simulink model "dPendDisUKF"  (Simulink 7.0)
settings: Solver=ode4  StartTime=0.0  StopTime=20  FixedStep=ts  RelTol=1e-3
InitFcn:
  | %dPendInit;
undefined symbols (not defined in the file): a, accel, B, b, c, c1, c2, d, g, l1, m, m1, m2, magnitude, n, p, P0, Qu, r1, r2, Ru, ts, W, WM, X0
libraries: simulink x4
settings Model: Creator=raje_ra  LastModifiedBy=vector  BufferReuse=off
settings OptimizationCC: OptimizeBlockIOStorage=off  BufferReuse=off  ExpressionFolding=off  LocalBlockOutputs=off

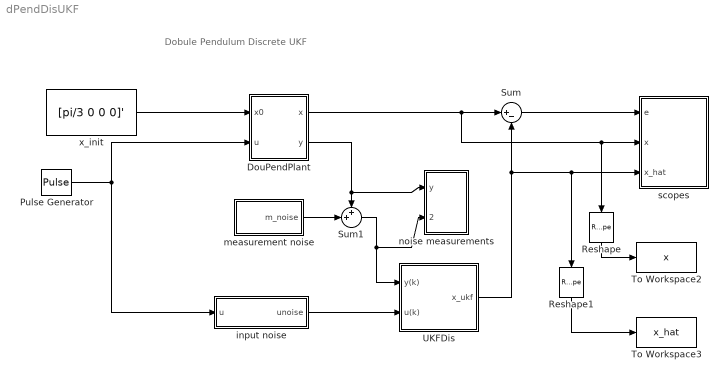
== system dPendDisUKF ==
  note: Dobule Pendulum Discrete UKF
  DouPendPlant : Subsystem
  Pulse Generator : DiscretePulseGenerator  PulseType=Time based  Amplitude=0.001  Period=1  PulseWidth=50
  Reshape : Reshape  Orientation=down
  Reshape1 : Reshape  Orientation=down
  Sum : Sum  Inputs=|+-  OutDataType=sfix(16)  OutScaling=2^0
  Sum1 : Sum  Inputs=++|  OutDataType=sfix(16)  OutScaling=2^0
  To Workspace2 : ToWorkspace  VariableName=x  SampleTime=-1  SaveFormat=Structure With Time
  To Workspace3 : ToWorkspace  VariableName=x_hat  SampleTime=-1  SaveFormat=Structure With Time
  UKFDis : Subsystem
  input noise : Subsystem
  measurement noise : Subsystem
  noise measurements : Subsystem
  scopes : Subsystem
  x_init : Constant  Value=[pi/3 0 0 0]'  VectorParams1D=off  OutDataType=sfix(16)  OutScaling=2^0
  wires:
  x_init/1 -> DouPendPlant/1(x0)
  DouPendPlant/1(x) -> Sum/1, scopes/2(x), Reshape/1
  UKFDis/1(x_ukf) -> Sum/2, scopes/3(x_hat), Reshape1/1
  Sum/1 -> scopes/1(e)
  Pulse Generator/1 -> DouPendPlant/2(u), input noise/1(u)
  DouPendPlant/2(y) -> Sum1/1, noise measurements/1(y)
  Sum1/1 -> UKFDis/1(y(k)), noise measurements/2(ynoise)
  measurement noise/1(m_noise) -> Sum1/2
  input noise/1(unoise) -> UKFDis/2(u(k))
  Reshape/1 -> To Workspace2/1
  Reshape1/1 -> To Workspace3/1

== system dPendDisUKF/DouPendPlant ==
  x0 : Inport
  u : Inport  Port=2
  F(x) : Subsystem
  Integrator1 : Integrator  InitialConditionSource=external  InitialCondition=[pi/3,-pi/3]'
  Measurements : Subsystem
  x : Outport  OutDataType=sfix(16)  OutScaling=2^0
  y : Outport  Port=2  OutDataType=sfix(16)  OutScaling=2^0
  wires:
  u/1 -> Measurements/2(u), F(x)/2(u)
  F(x)/1(x_dot) -> Integrator1/1
  Integrator1/1 -> x/1, F(x)/1(x), Measurements/1(x)  "x"
  x0/1 -> Integrator1/2
  Measurements/1(y) -> y/1

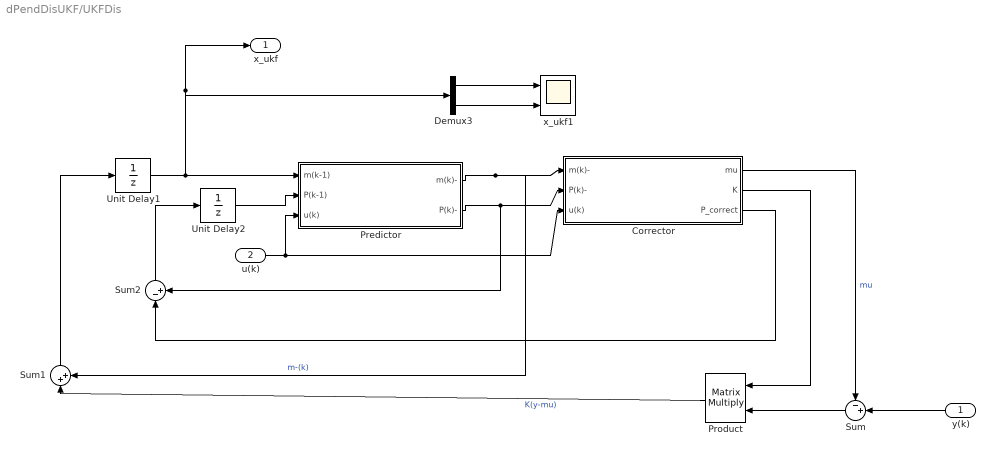
== system dPendDisUKF/UKFDis ==
  y(k) : Inport  Orientation=left
  u(k) : Inport  Port=2
  Corrector : Subsystem
  Demux3 : Demux  Outputs=2
  Predictor : Subsystem
  Product : Product  Orientation=left  Multiplication=Matrix(*)  OutDataType=sfix(16)  OutScaling=2^0  RndMeth=Zero
  Sum : Sum  Orientation=left  Inputs=-+|  OutDataType=sfix(16)  OutScaling=2^0
  Sum1 : Sum  Orientation=up  Inputs=|++  OutDataType=sfix(16)  OutScaling=2^0
  Sum2 : Sum  Orientation=up  Inputs=|-+  OutDataType=sfix(16)  OutScaling=2^0
  Unit Delay1 : UnitDelay  X0=X0  SampleTime=-1
  Unit Delay2 : UnitDelay  X0=P0  SampleTime=-1
  x_ukf1 : Scope  NumInputPorts=2
      settings: TimeRange=30  YMin=-15~-10  YMax=15~50  SaveName=ScopeData2
  x_ukf : Outport  OutDataType=sfix(16)  OutScaling=2^0
  wires:
  Sum2/1 -> Unit Delay2/1
  Corrector/3(P_correct) -> Sum2/1
  Unit Delay2/1 -> Predictor/2(P(k-1))
  Product/1 -> Sum1/1  "K(y-mu)"
  Sum/1 -> Product/2
  y(k)/1 -> Sum/2
  Corrector/2(K) -> Product/1
  Corrector/1(mu) -> Sum/1  "mu"
  Predictor/2(P(k)-) -> Sum2/2, Corrector/2(P(k)-)
  Predictor/1(m(k)-) -> Sum1/2, Corrector/1(m(k)-)  "m-(k)"
  Unit Delay1/1 -> Predictor/1(m(k-1)), x_ukf/1, Demux3/1
  Sum1/1 -> Unit Delay1/1
  Demux3/2 -> x_ukf1/2
  Demux3/1 -> x_ukf1/1
  u(k)/1 -> Predictor/3(u(k)), Corrector/3(u(k))

== system dPendDisUKF/input noise ==
  u : Inport
  Band-Limited White Noise : simulink/Sources/Band-Limited White Noise  SystemSampleTime=-1  Cov=[1e-6]  Ts=ts  seed=[23341]
  Sum2 : Sum  Inputs=++|  OutDataType=sfix(16)  OutScaling=2^0
  To Workspace2 : ToWorkspace  VariableName=Q_in  SampleTime=-1  SaveFormat=Array
  unoise : Outport
  wires:
  Sum2/1 -> unoise/1
  u/1 -> Sum2/2
  Band-Limited White Noise/1 -> To Workspace2/1, Sum2/1

== system dPendDisUKF/measurement noise ==
  Band-Limited White Noise - gyro : simulink/Sources/Band-Limited White Noise  SystemSampleTime=-1  Cov=[1e-7]  Ts=ts  seed=[23341]
  Band-Limited White Noise- q,dq : simulink/Sources/Band-Limited White Noise  SystemSampleTime=-1  Cov=[1e-9]  Ts=ts  seed=[23341]
  Band-Limited White Noise-IMU : simulink/Sources/Band-Limited White Noise  SystemSampleTime=-1  Cov=[1e-5]  Ts=ts  seed=[23341]
  Mux : Mux  Inputs=5
  To Workspace : ToWorkspace  VariableName=R_in  SampleTime=-1  SaveFormat=Array
  m_noise : Outport
  wires:
  Band-Limited White Noise-IMU/1 -> Mux/5, Mux/4
  Band-Limited White Noise - gyro/1 -> Mux/3
  Mux/1 -> To Workspace/1, m_noise/1
  Band-Limited White Noise- q,dq/1 -> Mux/2, Mux/1

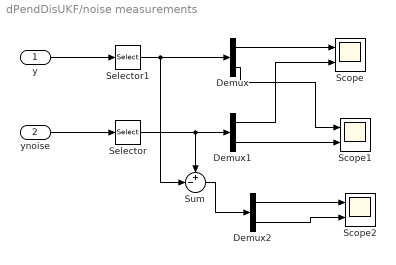
== system dPendDisUKF/noise measurements ==
  y : Inport
  ynoise : Inport  Port=2
  Demux : Demux  Outputs=2
  Demux1 : Demux  Outputs=2
  Demux2 : Demux  Outputs=2
  Scope : Scope  NumInputPorts=2
      settings: YMin=-60~-60  YMax=180~180
  Scope1 : Scope  NumInputPorts=2
      settings: YMin=-60~-60  YMax=180~180  SaveName=ScopeData5
  Scope2 : Scope  NumInputPorts=2
      settings: YMin=-60~-60  YMax=180~180  SaveName=ScopeData6
  Selector : Selector  InputPortWidth=5  IndexOptions=Index vector (dialog)  Indices=[1,2]  OutputSizes=1
  Selector1 : Selector  InputPortWidth=5  IndexOptions=Index vector (dialog)  Indices=[1,2]  OutputSizes=1
  Sum : Sum  Inputs=+-|  OutDataType=sfix(16)  OutScaling=2^0
  wires:
  Demux2/2 -> Scope2/2
  Demux2/1 -> Scope2/1
  Demux1/2 -> Scope1/2
  Demux/2 -> Scope1/1
  Demux1/1 -> Scope/2
  Demux/1 -> Scope/1
  Sum/1 -> Demux2/1
  Selector/1 -> Sum/1, Demux1/1
  Selector1/1 -> Sum/2, Demux/1
  ynoise/1 -> Selector/1
  y/1 -> Selector1/1

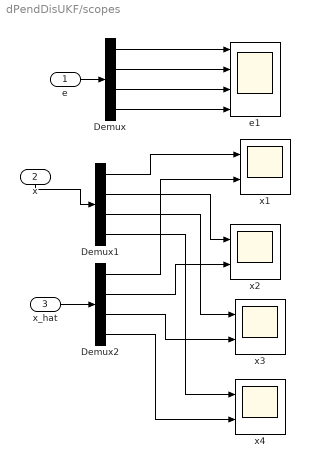
== system dPendDisUKF/scopes ==
  e : Inport
  x : Inport  Orientation=down  Port=2
  x_hat : Inport  Port=3
  Demux : Demux
  Demux1 : Demux
  Demux2 : Demux
  e1 : Scope  NumInputPorts=4
      settings: TickLabels=on  YMin=-30~-20~-120~-17.5  YMax=80~27.5~20~25
  x{1..4} (4 alike) : Scope  NumInputPorts=2
      x1 settings: TickLabels=on  YMin=-5~-5  YMax=14~22.5  SaveName=ScopeData3
      x2 settings: TickLabels=on  YMin=-11~-11  YMax=11~11  SaveName=ScopeData4
      x3 settings: TickLabels=on  YMin=-10~-10  YMax=27.5~27.5  SaveName=ScopeData7
      x4 settings: TickLabels=on  YMin=-15~-15  YMax=12.5~12.5  SaveName=ScopeData8
  wires:
  e/1 -> Demux/1
  x_hat/1 -> Demux2/1
  x/1 -> Demux1/1
  Demux2/4 -> x4/2
  Demux1/4 -> x4/1
  Demux2/3 -> x3/2
  Demux1/3 -> x3/1
  Demux2/2 -> x2/2
  Demux1/2 -> x2/1
  Demux2/1 -> x1/2
  Demux1/1 -> x1/1
  Demux/4 -> e1/4
  Demux/3 -> e1/3
  Demux/2 -> e1/2
  Demux/1 -> e1/1

== system dPendDisUKF/DouPendPlant/F(x) ==
  x : Inport
  u : Inport  Port=2
  Add : Sum  Inputs=+++  OutDataType=sfix(16)  OutScaling=2^-10
  Divide : Product  Inputs=/*  Multiplication=Matrix(*)  OutDataType=sfix(16)  OutScaling=2^-10
  Gain : Gain  Gain=diag([0,c1,0,c2])  Multiplication=Matrix(K*u)  ParameterDataType=sfix(16)  ParameterScaling=2^0  OutDataType=sfix(16)  OutScaling=2^0
  Gain1 : Gain  Gain=B  ParameterDataType=sfix(16)  ParameterScaling=2^0  OutDataType=sfix(16)  OutScaling=2^0
  M matrix : Subsystem
  h+g : Subsystem
  x_dot : Outport
  wires:
  x/1 -> M matrix/1(x), h+g/1(x), Gain/1
  h+g/1(-(h+g)) -> Add/1
  Gain/1 -> Add/2
  u/1 -> Gain1/1
  Add/1 -> Divide/2
  Gain1/1 -> Add/3
  M matrix/1(M) -> Divide/1
  Divide/1 -> x_dot/1

== system dPendDisUKF/DouPendPlant/Measurements ==
  x : Inport
  u : Inport  Port=2
  Display : Display
  IMU : Subsystem
  Mux : Mux  Inputs=3
  Selector1 : Selector  InputPortWidth=4  IndexOptions=Index vector (dialog)  Indices=[3 4]  OutputSizes=1
  Selector2 : Selector  InputPortWidth=4  IndexOptions=Index vector (dialog)  Indices=[2 4]  OutputSizes=1
  Sum of Elements : Sum  Inputs=+  OutDataType=sfix(16)  OutScaling=2^-10
  y : Outport  OutDataType=sfix(16)  OutScaling=2^0
  wires:
  IMU/1(acc) -> Mux/3
  u/1 -> IMU/2(u(k))
  Sum of Elements/1 -> Mux/2  "(dq_1+dq_2)"
  Selector2/1 -> Sum of Elements/1
  Mux/1 -> Display/1, y/1
  Selector1/1 -> Mux/1
  x/1 -> IMU/1(m(k)-), Selector2/1, Selector1/1

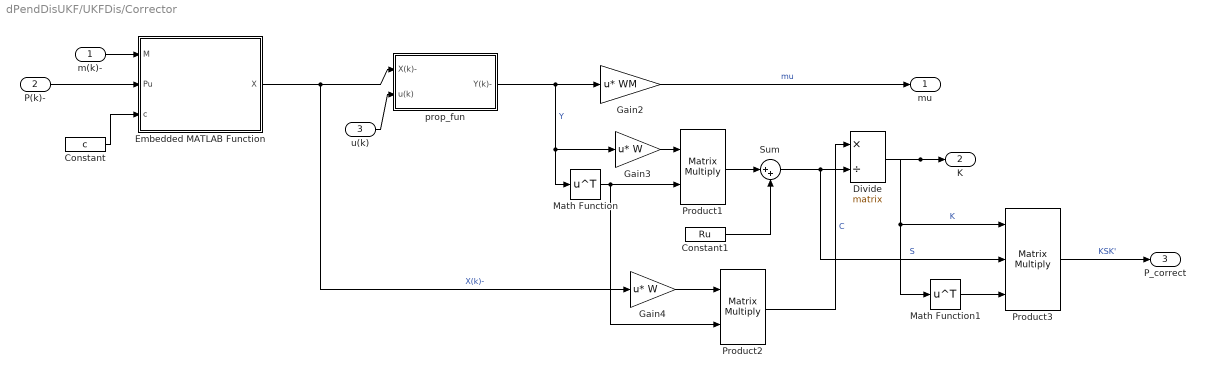
== system dPendDisUKF/UKFDis/Corrector ==
  m(k)- : Inport
  P(k)- : Inport  Port=2
  u(k) : Inport  Port=3
  Constant : Constant  Value=c  OutDataType=sfix(16)  OutScaling=2^0
  Constant1 : Constant  Value=Ru  OutDataType=sfix(16)  OutScaling=2^0
  Divide : Product  Inputs=*/  Multiplication=Matrix(*)  OutDataType=sfix(16)  OutScaling=2^-10
  Embedded MATLAB Function : Stateflow chart
  Gain2 : Gain  Gain=WM  Multiplication=Matrix(u*K)  ParameterDataType=sfix(16)  ParameterScaling=2^0  OutDataType=sfix(16)  OutScaling=2^0
  Gain3 : Gain  Gain=W  Multiplication=Matrix(u*K)  ParameterDataType=sfix(16)  ParameterScaling=2^0  OutDataType=sfix(16)  OutScaling=2^0
  Gain4 : Gain  Gain=W  Multiplication=Matrix(u*K)  ParameterDataType=sfix(16)  ParameterScaling=2^0  OutDataType=sfix(16)  OutScaling=2^0
  Math Function : Math  Operator=transpose  OutDataType=sfix(16)  OutScaling=2^0  SaturateOnIntegerOverflow=on
  Math Function1 : Math  Operator=transpose  OutDataType=sfix(16)  OutScaling=2^0  SaturateOnIntegerOverflow=on
  Product1 : Product  Multiplication=Matrix(*)  OutDataType=sfix(16)  OutScaling=2^0  RndMeth=Zero
  Product2 : Product  Multiplication=Matrix(*)  OutDataType=sfix(16)  OutScaling=2^0  RndMeth=Zero
  Product3 : Product  Inputs=3  Multiplication=Matrix(*)  OutDataType=sfix(16)  OutScaling=2^0  RndMeth=Zero
  Sum : Sum  Inputs=|++  OutDataType=sfix(16)  OutScaling=2^0
  prop_fun : Subsystem
  mu : Outport
  K : Outport  Port=2
  P_correct : Outport  Port=3
  wires:
  Product3/1 -> P_correct/1  "KSK'"
  Math Function1/1 -> Product3/3
  Divide/1 -> Math Function1/1, Product3/1, K/1  "K"
  Sum/1 -> Product3/2, Divide/2  "S"
  Product2/1 -> Divide/1  "C"
  Gain4/1 -> Product2/1
  Constant1/1 -> Sum/2
  Product1/1 -> Sum/1
  Math Function/1 -> Product2/2, Product1/2
  Gain3/1 -> Product1/1
  Gain2/1 -> mu/1  "mu"
  prop_fun/1(Y(k)-) -> Math Function/1, Gain3/1, Gain2/1  "Y"
  Embedded MATLAB Function/1(X) -> Gain4/1, prop_fun/1(X(k)-)  "X(k)-"
  Constant/1 -> Embedded MATLAB Function/3(c)
  P(k)-/1 -> Embedded MATLAB Function/2(Pu)
  m(k)-/1 -> Embedded MATLAB Function/1(M)
  u(k)/1 -> prop_fun/2(u(k))

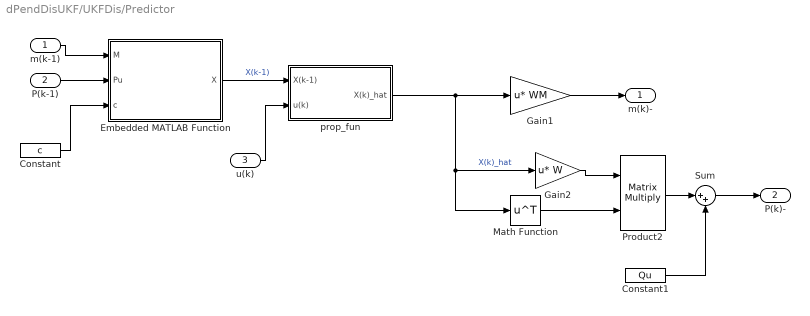
== system dPendDisUKF/UKFDis/Predictor ==
  m(k-1) : Inport
  P(k-1) : Inport  Port=2
  u(k) : Inport  Port=3
  Constant : Constant  Value=c  OutDataType=sfix(16)  OutScaling=2^0
  Constant1 : Constant  Value=Qu  OutDataType=sfix(16)  OutScaling=2^0
  Embedded MATLAB Function : Stateflow chart
  Gain1 : Gain  Gain=WM  Multiplication=Matrix(u*K)  ParameterDataType=sfix(16)  ParameterScaling=2^0  OutDataType=sfix(16)  OutScaling=2^0
  Gain2 : Gain  Gain=W  Multiplication=Matrix(u*K)  ParameterDataType=sfix(16)  ParameterScaling=2^0  OutDataType=sfix(16)  OutScaling=2^0
  Math Function : Math  Operator=transpose  OutDataType=sfix(16)  OutScaling=2^0  SaturateOnIntegerOverflow=on
  Product2 : Product  Multiplication=Matrix(*)  OutDataType=sfix(16)  OutScaling=2^0  RndMeth=Zero
  Sum : Sum  Inputs=|++  OutDataType=sfix(16)  OutScaling=2^0
  prop_fun : Subsystem
  m(k)- : Outport
  P(k)- : Outport  Port=2
  wires:
  prop_fun/1(X(k)_hat) -> Gain1/1, Math Function/1, Gain2/1  "X(k)_hat"
  Gain1/1 -> m(k)-/1
  P(k-1)/1 -> Embedded MATLAB Function/2(Pu)
  m(k-1)/1 -> Embedded MATLAB Function/1(M)
  Constant/1 -> Embedded MATLAB Function/3(c)
  Sum/1 -> P(k)-/1
  Constant1/1 -> Sum/2
  Product2/1 -> Sum/1
  Math Function/1 -> Product2/2
  Gain2/1 -> Product2/1
  Embedded MATLAB Function/1(X) -> prop_fun/1(X(k-1))  "X(k-1)"
  u(k)/1 -> prop_fun/2(u(k))

== system dPendDisUKF/DouPendPlant/F(x)/M matrix ==
  x : Inport
  M1 : Constant  Value=[1,0,0,0]  VectorParams1D=off  OutDataType=sfix(16)  OutScaling=2^0
  M2 : Subsystem
  M3 : Constant  Value=[0,0,1,0]  VectorParams1D=off  OutDataType=sfix(16)  OutScaling=2^0
  M4 : Subsystem
  Matrix Concatenate : Concatenate  NumInputs=4  Mode=Multidimensional array
  Selector : Selector  InputPortWidth=4  IndexOptions=Index vector (dialog)  Indices=[3]  OutputSizes=1
  M : Outport
  wires:
  Selector/1 -> M2/1(x3), M4/1(x3)  "x3"
  M1/1 -> Matrix Concatenate/1
  M2/1(Out1) -> Matrix Concatenate/2
  M3/1 -> Matrix Concatenate/3
  M4/1(Out) -> Matrix Concatenate/4
  x/1 -> Selector/1
  Matrix Concatenate/1 -> M/1

== system dPendDisUKF/DouPendPlant/F(x)/h+g ==
  x : Inport
  Selector : Selector  InputPortWidth=4  IndexOptions=Index vector (dialog)  Indices=[2]  OutputSizes=1
  Selector1 : Selector  InputPortWidth=4  IndexOptions=Index vector (dialog)  Indices=[4]  OutputSizes=1
  Vector Concatenate : Concatenate  NumInputs=4  Mode=Vector
  h+g(2) : Subsystem
  h+g(4) : Subsystem
  -(h+g) : Outport
  wires:
  x/1 -> Selector/1, h+g(2)/1(x), Selector1/1, h+g(4)/1(x)
  Selector/1 -> Vector Concatenate/1  "x2"
  h+g(2)/1(-F(1)) -> Vector Concatenate/2
  Selector1/1 -> Vector Concatenate/3
  h+g(4)/1(-F(2)) -> Vector Concatenate/4
  Vector Concatenate/1 -> -(h+g)/1

== system dPendDisUKF/DouPendPlant/Measurements/IMU ==
  m(k)- : Inport
  u(k) : Inport  Port=2
  Mux : Mux  Inputs=2
  Transpose : Math  Operator=transpose  OutDataType=sfix(16)  OutScaling=2^0  SaturateOnIntegerOverflow=on
  acceleration : MATLABFcn  MATLABFcn=accel(u,p)  Output1D=off
  acc : Outport
  wires:
  u(k)/1 -> Mux/2
  acceleration/1 -> acc/1  "acc"
  m(k)-/1 -> Mux/1
  Transpose/1 -> acceleration/1
  Mux/1 -> Transpose/1

== system dPendDisUKF/UKFDis/Corrector/prop_fun ==
  X(k)- : Inport
  u(k) : Inport  Port=2
  F(X) : Subsystem  TreatAsAtomicUnit=on
  Y(k)- : Outport
  wires:
  F(X)/1(Y(k)-) -> Y(k)-/1
  X(k)-/1 -> F(X)/1(X(k)-)
  u(k)/1 -> F(X)/2(u(k))

== system dPendDisUKF/UKFDis/Predictor/prop_fun ==
  X(k-1) : Inport
  u(k) : Inport  Port=2
  F(X) : Subsystem  TreatAsAtomicUnit=on
  Gain3 : Gain  Gain=ts  ParameterDataType=sfix(16)  ParameterScaling=2^0  OutDataType=sfix(16)  OutScaling=2^0
  Sum1 : Sum  Inputs=|++  OutDataType=sfix(16)  OutScaling=2^0
  X(k)_hat : Outport
  wires:
  Gain3/1 -> Sum1/1
  F(X)/1(F(X)) -> Gain3/1
  X(k-1)/1 -> F(X)/1(X(k-1)), Sum1/2
  Sum1/1 -> X(k)_hat/1
  u(k)/1 -> F(X)/2(u(k))

== system dPendDisUKF/DouPendPlant/F(x)/M matrix/M2 ==
  x3 : Inport
  M21 : Constant  Value=0  VectorParams1D=off  OutDataType=sfix(16)  OutScaling=2^0
  M22 : Subsystem
  M23 : Constant  Value=0  VectorParams1D=off  OutDataType=sfix(16)  OutScaling=2^0
  M24 : Subsystem
  Math Function : Math  Operator=transpose  OutDataType=sfix(16)  OutScaling=2^0  SaturateOnIntegerOverflow=on
  Vector Concatenate : Concatenate  NumInputs=4  Mode=Vector
  Out1 : Outport
  wires:
  x3/1 -> M22/1(x3), M24/1(x3)
  M21/1 -> Vector Concatenate/1
  M22/1(M22) -> Vector Concatenate/2
  M23/1 -> Vector Concatenate/3
  M24/1(M24) -> Vector Concatenate/4
  Vector Concatenate/1 -> Math Function/1
  Math Function/1 -> Out1/1

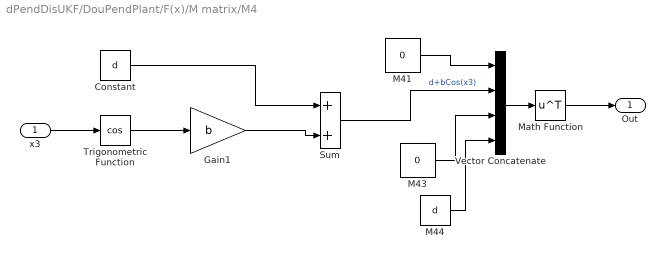
== system dPendDisUKF/DouPendPlant/F(x)/M matrix/M4 ==
  x3 : Inport
  Constant : Constant  Value=d  OutDataType=sfix(16)  OutScaling=2^0
  Gain1 : Gain  Gain=b  ParameterDataType=sfix(16)  ParameterScaling=2^0  OutDataType=sfix(16)  OutScaling=2^0
  M41 : Constant  Value=0  VectorParams1D=off  OutDataType=sfix(16)  OutScaling=2^0
  M43 : Constant  Value=0  VectorParams1D=off  OutDataType=sfix(16)  OutScaling=2^0
  M44 : Constant  Value=d  OutDataType=sfix(16)  OutScaling=2^0
  Math Function : Math  Operator=transpose  OutDataType=sfix(16)  OutScaling=2^0  SaturateOnIntegerOverflow=on
  Sum : Sum  OutDataType=sfix(16)  OutScaling=2^0
  Trigonometric Function : Trigonometry  Operator=cos
  Vector Concatenate : Concatenate  NumInputs=4  Mode=Vector
  Out : Outport
  wires:
  x3/1 -> Trigonometric Function/1
  Gain1/1 -> Sum/2
  Trigonometric Function/1 -> Gain1/1
  M41/1 -> Vector Concatenate/1
  Sum/1 -> Vector Concatenate/2  "d+bCos(x3)"
  M44/1 -> Vector Concatenate/4
  M43/1 -> Vector Concatenate/3
  Vector Concatenate/1 -> Math Function/1
  Math Function/1 -> Out/1
  Constant/1 -> Sum/1

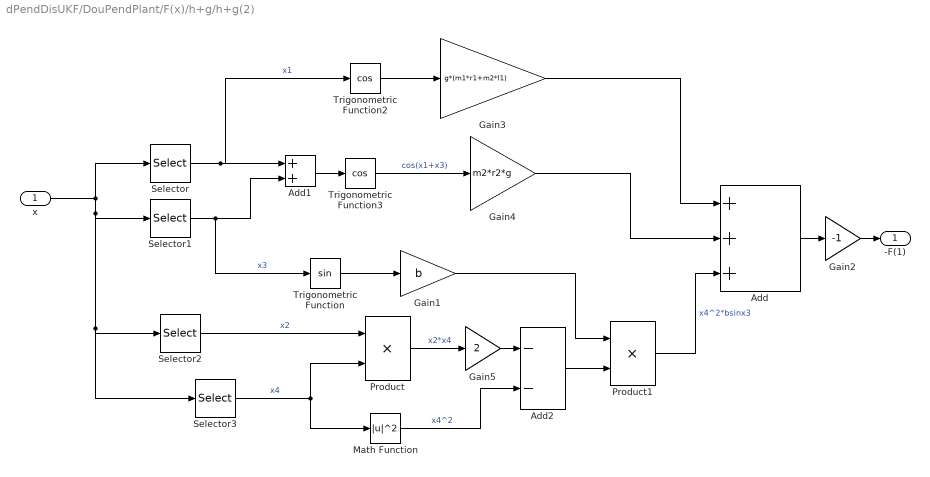
== system dPendDisUKF/DouPendPlant/F(x)/h+g/h+g(2) ==
  x : Inport
  Add : Sum  Inputs=+++  OutDataType=sfix(16)  OutScaling=2^-10
  Add1 : Sum  OutDataType=sfix(16)  OutScaling=2^-10
  Add2 : Sum  Inputs=--  OutDataType=sfix(16)  OutScaling=2^-10
  Gain1 : Gain  Gain=b  ParameterDataType=sfix(16)  ParameterScaling=2^0  OutDataType=sfix(16)  OutScaling=2^0
  Gain2 : Gain  Gain=-1  ParameterDataType=sfix(16)  ParameterScaling=2^0  OutDataType=sfix(16)  OutScaling=2^0
  Gain3 : Gain  Gain=g*(m1*r1+m2*l1)  ParameterDataType=sfix(16)  ParameterScaling=2^0  OutDataType=sfix(16)  OutScaling=2^0
  Gain4 : Gain  Gain=m2*r2*g  ParameterDataType=sfix(16)  ParameterScaling=2^0  OutDataType=sfix(16)  OutScaling=2^0
  Gain5 : Gain  Gain=2  ParameterDataType=sfix(16)  ParameterScaling=2^0  OutDataType=sfix(16)  OutScaling=2^0
  Math Function : Math  Operator=magnitude^2  OutDataType=sfix(16)  OutScaling=2^0  SaturateOnIntegerOverflow=on
  Product : Product  OutDataType=sfix(16)  OutScaling=2^0  RndMeth=Zero
  Product1 : Product  OutDataType=sfix(16)  OutScaling=2^0  RndMeth=Zero
  Selector : Selector  InputPortWidth=4  IndexOptions=Index vector (dialog)  Indices=[1]  OutputSizes=1
  Selector1 : Selector  InputPortWidth=4  IndexOptions=Index vector (dialog)  Indices=[3]  OutputSizes=1
  Selector2 : Selector  InputPortWidth=4  IndexOptions=Index vector (dialog)  Indices=[2]  OutputSizes=1
  Selector3 : Selector  InputPortWidth=4  IndexOptions=Index vector (dialog)  Indices=[4]  OutputSizes=1
  Trigonometric Function : Trigonometry
  Trigonometric Function2 : Trigonometry  Operator=cos
  Trigonometric Function3 : Trigonometry  Operator=cos
  -F(1) : Outport  OutDataType=sfix(16)  OutScaling=2^0
  wires:
  Trigonometric Function/1 -> Gain1/1
  Selector1/1 -> Add1/2, Trigonometric Function/1  "x3"
  Selector/1 -> Add1/1, Trigonometric Function2/1  "x1"
  Trigonometric Function2/1 -> Gain3/1
  Gain3/1 -> Add/1
  Trigonometric Function3/1 -> Gain4/1  "cos(x1+x3)"
  Add1/1 -> Trigonometric Function3/1
  Gain4/1 -> Add/2
  Product1/1 -> Add/3  "x4^2*bsinx3"
  Add/1 -> Gain2/1
  x/1 -> Selector/1, Selector1/1, Selector2/1, Selector3/1
  Selector3/1 -> Product/2, Math Function/1  "x4"
  Selector2/1 -> Product/1  "x2"
  Math Function/1 -> Add2/2  "x4^2"
  Product/1 -> Gain5/1  "x2*x4"
  Gain5/1 -> Add2/1
  Add2/1 -> Product1/2
  Gain1/1 -> Product1/1
  Gain2/1 -> -F(1)/1

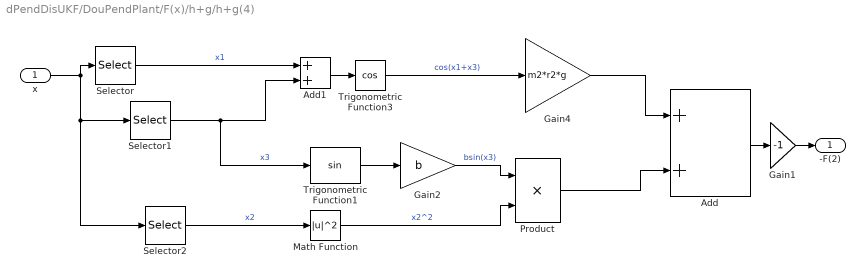
== system dPendDisUKF/DouPendPlant/F(x)/h+g/h+g(4) ==
  x : Inport
  Add : Sum  OutDataType=sfix(16)  OutScaling=2^-10
  Add1 : Sum  OutDataType=sfix(16)  OutScaling=2^-10
  Gain1 : Gain  Gain=-1  ParameterDataType=sfix(16)  ParameterScaling=2^0  OutDataType=sfix(16)  OutScaling=2^0
  Gain2 : Gain  Gain=b  ParameterDataType=sfix(16)  ParameterScaling=2^0  OutDataType=sfix(16)  OutScaling=2^0
  Gain4 : Gain  Gain=m2*r2*g  ParameterDataType=sfix(16)  ParameterScaling=2^0  OutDataType=sfix(16)  OutScaling=2^0
  Math Function : Math  Operator=magnitude^2  OutDataType=sfix(16)  OutScaling=2^0  SaturateOnIntegerOverflow=on
  Product : Product  OutDataType=sfix(16)  OutScaling=2^0  RndMeth=Zero
  Selector : Selector  InputPortWidth=4  IndexOptions=Index vector (dialog)  Indices=[1]  OutputSizes=1
  Selector1 : Selector  InputPortWidth=4  IndexOptions=Index vector (dialog)  Indices=[3]  OutputSizes=1
  Selector2 : Selector  InputPortWidth=4  IndexOptions=Index vector (dialog)  Indices=[2]  OutputSizes=1
  Trigonometric Function1 : Trigonometry
  Trigonometric Function3 : Trigonometry  Operator=cos
  -F(2) : Outport  OutDataType=sfix(16)  OutScaling=2^0
  wires:
  Selector2/1 -> Math Function/1  "x2"
  Product/1 -> Add/2
  Gain4/1 -> Add/1
  x/1 -> Selector/1, Selector1/1, Selector2/1
  Trigonometric Function1/1 -> Gain2/1
  Selector1/1 -> Trigonometric Function1/1, Add1/2  "x3"
  Selector/1 -> Add1/1  "x1"
  Trigonometric Function3/1 -> Gain4/1  "cos(x1+x3)"
  Add1/1 -> Trigonometric Function3/1
  Add/1 -> Gain1/1
  Gain2/1 -> Product/1  "bsin(x3)"
  Math Function/1 -> Product/2  "x2^2"
  Gain1/1 -> -F(2)/1

== system dPendDisUKF/UKFDis/Corrector/prop_fun/F(X) ==
  X(k)- : Inport  OutDataType=sfix(16)  OutScaling=2^0
  u(k) : Inport  Port=2  OutDataType=sfix(16)  OutScaling=2^0
  Assignment : Assignment  NumberOfDimensions=2  IndexOptions=Assign all,Index vector (port)  Indices=1,1  OutputSizes=2,2
  Constant : Constant  Value=zeros(m,2*n+1)  VectorParams1D=off  OutDataType=sfix(16)  OutScaling=2^0  SampleTime=-1
  Display : Display
  For Iterator : ForIterator  ResetStates=reset  IterationLimit=2*n +1  IterationVariableDataType=double
  Measurements : Subsystem
  Selector : Selector  NumberOfDimensions=2  IndexOptions=Select all,Index vector (port)  Indices=[1 3],1  OutputSizes=1,1
  Y(k)- : Outport  OutDataType=sfix(16)  OutScaling=2^0
  wires:
  X(k)-/1 -> Selector/1
  For Iterator/1 -> Selector/2, Assignment/3, Display/1
  Selector/1 -> Measurements/1(x)
  Measurements/1(y) -> Assignment/2
  Assignment/1 -> Y(k)-/1
  Constant/1 -> Assignment/1
  u(k)/1 -> Measurements/2(u)

== system dPendDisUKF/UKFDis/Predictor/prop_fun/F(X) ==
  X(k-1) : Inport  OutDataType=sfix(16)  OutScaling=2^0
  u(k) : Inport  Port=2  OutDataType=sfix(16)  OutScaling=2^0
  Assignment : Assignment  NumberOfDimensions=2  IndexOptions=Assign all,Index vector (port)  Indices=1,1  OutputSizes=2,2
  F(x) : Subsystem
  For Iterator : ForIterator  ResetStates=reset  IterationLimit=2*n +1  IterationVariableDataType=double
  Selector : Selector  NumberOfDimensions=2  IndexOptions=Select all,Index vector (port)  Indices=[1 3],1  OutputSizes=1,1
  F(X) : Outport  OutDataType=sfix(16)  OutScaling=2^0
  wires:
  X(k-1)/1 -> Selector/1, Assignment/1
  For Iterator/1 -> Selector/2, Assignment/3
  Selector/1 -> F(x)/1(x)
  F(x)/1(x_dot) -> Assignment/2
  Assignment/1 -> F(X)/1
  u(k)/1 -> F(x)/2(u)

== system dPendDisUKF/DouPendPlant/F(x)/M matrix/M2/M22 ==
  x3 : Inport
  Constant : Constant  Value=a  OutDataType=sfix(16)  OutScaling=2^0
  Gain1 : Gain  Gain=2*b  ParameterDataType=sfix(16)  ParameterScaling=2^0  OutDataType=sfix(16)  OutScaling=2^0
  Sum : Sum  OutDataType=sfix(16)  OutScaling=2^0
  Trigonometric Function : Trigonometry  Operator=cos
  M22 : Outport
  wires:
  x3/1 -> Trigonometric Function/1
  Sum/1 -> M22/1  "a+2bCos(x3)"
  Gain1/1 -> Sum/2
  Trigonometric Function/1 -> Gain1/1
  Constant/1 -> Sum/1

== system dPendDisUKF/DouPendPlant/F(x)/M matrix/M2/M24 ==
  x3 : Inport
  Constant : Constant  Value=d  OutDataType=sfix(16)  OutScaling=2^0
  Gain1 : Gain  Gain=b  ParameterDataType=sfix(16)  ParameterScaling=2^0  OutDataType=sfix(16)  OutScaling=2^0
  Sum : Sum  OutDataType=sfix(16)  OutScaling=2^0
  Trigonometric Function : Trigonometry  Operator=cos
  M24 : Outport
  wires:
  Trigonometric Function/1 -> Gain1/1
  Gain1/1 -> Sum/2
  Sum/1 -> M24/1  "d+bCos(x3)"
  x3/1 -> Trigonometric Function/1
  Constant/1 -> Sum/1

== system dPendDisUKF/UKFDis/Corrector/prop_fun/F(X)/Measurements ==
  x : Inport
  u : Inport  Port=2
  Display : Display
  IMU : Subsystem
  Mux : Mux  Inputs=3
  Selector1 : Selector  InputPortWidth=4  IndexOptions=Index vector (dialog)  Indices=[3 4]  OutputSizes=1
  Selector2 : Selector  InputPortWidth=4  IndexOptions=Index vector (dialog)  Indices=[2 4]  OutputSizes=1
  Sum of Elements : Sum  Inputs=+  OutDataType=sfix(16)  OutScaling=2^-10
  y : Outport  OutDataType=sfix(16)  OutScaling=2^0
  wires:
  IMU/1(acc) -> Mux/3
  u/1 -> IMU/2(u(k))
  Sum of Elements/1 -> Mux/2  "(dq_1+dq_2)"
  Selector2/1 -> Sum of Elements/1
  Mux/1 -> Display/1, y/1
  Selector1/1 -> Mux/1
  x/1 -> IMU/1(m(k)-), Selector2/1, Selector1/1

== system dPendDisUKF/UKFDis/Predictor/prop_fun/F(X)/F(x) ==
  x : Inport
  u : Inport  Port=2
  Add : Sum  Inputs=+++  OutDataType=sfix(16)  OutScaling=2^-10
  Divide : Product  Inputs=/*  Multiplication=Matrix(*)  OutDataType=sfix(16)  OutScaling=2^-10
  Gain : Gain  Gain=diag([0,c1,0,c2])  Multiplication=Matrix(K*u)  ParameterDataType=sfix(16)  ParameterScaling=2^0  OutDataType=sfix(16)  OutScaling=2^0
  Gain1 : Gain  Gain=B  ParameterDataType=sfix(16)  ParameterScaling=2^0  OutDataType=sfix(16)  OutScaling=2^0
  M matrix : Subsystem
  h+g : Subsystem
  x_dot : Outport
  wires:
  x/1 -> M matrix/1(x), h+g/1(x), Gain/1
  h+g/1(-(h+g)) -> Add/1
  Gain/1 -> Add/2
  u/1 -> Gain1/1
  Add/1 -> Divide/2
  Gain1/1 -> Add/3
  M matrix/1(M) -> Divide/1
  Divide/1 -> x_dot/1

== system dPendDisUKF/UKFDis/Corrector/prop_fun/F(X)/Measurements/IMU ==
  m(k)- : Inport
  u(k) : Inport  Port=2
  Mux : Mux  Inputs=2
  Transpose : Math  Operator=transpose  OutDataType=sfix(16)  OutScaling=2^0  SaturateOnIntegerOverflow=on
  acceleration : MATLABFcn  MATLABFcn=accel(u,p)  Output1D=off
  acc : Outport
  wires:
  u(k)/1 -> Mux/2
  acceleration/1 -> acc/1  "acc"
  m(k)-/1 -> Mux/1
  Transpose/1 -> acceleration/1
  Mux/1 -> Transpose/1

== system dPendDisUKF/UKFDis/Predictor/prop_fun/F(X)/F(x)/M matrix ==
  x : Inport
  M1 : Constant  Value=[1,0,0,0]  VectorParams1D=off  OutDataType=sfix(16)  OutScaling=2^0
  M2 : Subsystem
  M3 : Constant  Value=[0,0,1,0]  VectorParams1D=off  OutDataType=sfix(16)  OutScaling=2^0
  M4 : Subsystem
  Matrix Concatenate : Concatenate  NumInputs=4  Mode=Multidimensional array
  Selector : Selector  InputPortWidth=4  IndexOptions=Index vector (dialog)  Indices=[3]  OutputSizes=1
  M : Outport
  wires:
  Selector/1 -> M2/1(x3), M4/1(x3)  "x3"
  M1/1 -> Matrix Concatenate/1
  M2/1(Out1) -> Matrix Concatenate/2
  M3/1 -> Matrix Concatenate/3
  M4/1(Out) -> Matrix Concatenate/4
  x/1 -> Selector/1
  Matrix Concatenate/1 -> M/1

== system dPendDisUKF/UKFDis/Predictor/prop_fun/F(X)/F(x)/h+g ==
  x : Inport
  Selector : Selector  InputPortWidth=4  IndexOptions=Index vector (dialog)  Indices=[2]  OutputSizes=1
  Selector1 : Selector  InputPortWidth=4  IndexOptions=Index vector (dialog)  Indices=[4]  OutputSizes=1
  Vector Concatenate : Concatenate  NumInputs=4  Mode=Vector
  h+g(2) : Subsystem
  h+g(4) : Subsystem
  -(h+g) : Outport
  wires:
  x/1 -> Selector/1, h+g(2)/1(x), Selector1/1, h+g(4)/1(x)
  Selector/1 -> Vector Concatenate/1  "x2"
  h+g(2)/1(-F(1)) -> Vector Concatenate/2
  Selector1/1 -> Vector Concatenate/3
  h+g(4)/1(-F(2)) -> Vector Concatenate/4
  Vector Concatenate/1 -> -(h+g)/1

== system dPendDisUKF/UKFDis/Predictor/prop_fun/F(X)/F(x)/M matrix/M2 ==
  x3 : Inport
  M21 : Constant  Value=0  VectorParams1D=off  OutDataType=sfix(16)  OutScaling=2^0
  M22 : Subsystem
  M23 : Constant  Value=0  VectorParams1D=off  OutDataType=sfix(16)  OutScaling=2^0
  M24 : Subsystem
  Math Function : Math  Operator=transpose  OutDataType=sfix(16)  OutScaling=2^0  SaturateOnIntegerOverflow=on
  Vector Concatenate : Concatenate  NumInputs=4  Mode=Vector
  Out1 : Outport
  wires:
  x3/1 -> M22/1(x3), M24/1(x3)
  M21/1 -> Vector Concatenate/1
  M22/1(M22) -> Vector Concatenate/2
  M23/1 -> Vector Concatenate/3
  M24/1(M24) -> Vector Concatenate/4
  Vector Concatenate/1 -> Math Function/1
  Math Function/1 -> Out1/1

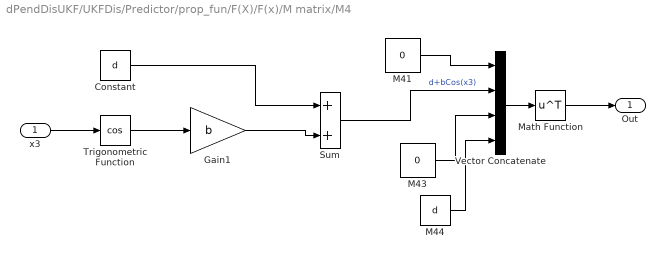
== system dPendDisUKF/UKFDis/Predictor/prop_fun/F(X)/F(x)/M matrix/M4 ==
  x3 : Inport
  Constant : Constant  Value=d  OutDataType=sfix(16)  OutScaling=2^0
  Gain1 : Gain  Gain=b  ParameterDataType=sfix(16)  ParameterScaling=2^0  OutDataType=sfix(16)  OutScaling=2^0
  M41 : Constant  Value=0  VectorParams1D=off  OutDataType=sfix(16)  OutScaling=2^0
  M43 : Constant  Value=0  VectorParams1D=off  OutDataType=sfix(16)  OutScaling=2^0
  M44 : Constant  Value=d  OutDataType=sfix(16)  OutScaling=2^0
  Math Function : Math  Operator=transpose  OutDataType=sfix(16)  OutScaling=2^0  SaturateOnIntegerOverflow=on
  Sum : Sum  OutDataType=sfix(16)  OutScaling=2^0
  Trigonometric Function : Trigonometry  Operator=cos
  Vector Concatenate : Concatenate  NumInputs=4  Mode=Vector
  Out : Outport
  wires:
  x3/1 -> Trigonometric Function/1
  Gain1/1 -> Sum/2
  Trigonometric Function/1 -> Gain1/1
  M41/1 -> Vector Concatenate/1
  Sum/1 -> Vector Concatenate/2  "d+bCos(x3)"
  M44/1 -> Vector Concatenate/4
  M43/1 -> Vector Concatenate/3
  Vector Concatenate/1 -> Math Function/1
  Math Function/1 -> Out/1
  Constant/1 -> Sum/1

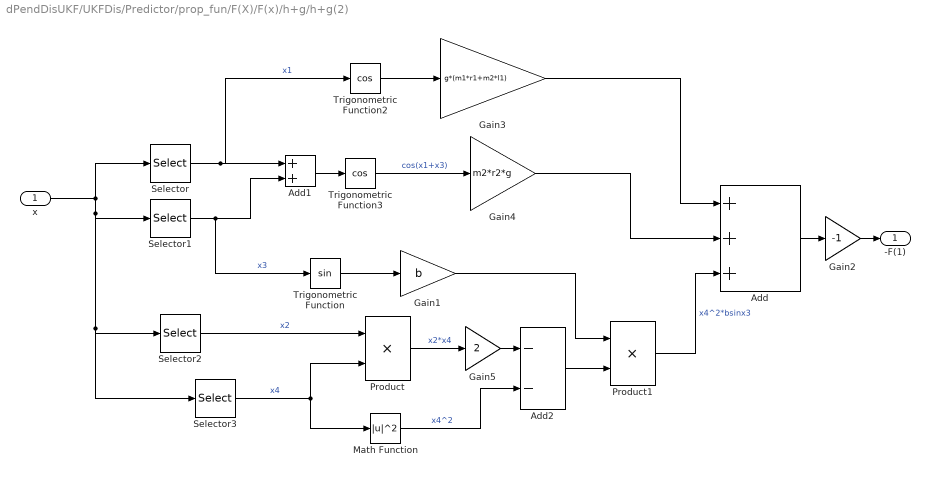
== system dPendDisUKF/UKFDis/Predictor/prop_fun/F(X)/F(x)/h+g/h+g(2) ==
  x : Inport
  Add : Sum  Inputs=+++  OutDataType=sfix(16)  OutScaling=2^-10
  Add1 : Sum  OutDataType=sfix(16)  OutScaling=2^-10
  Add2 : Sum  Inputs=--  OutDataType=sfix(16)  OutScaling=2^-10
  Gain1 : Gain  Gain=b  ParameterDataType=sfix(16)  ParameterScaling=2^0  OutDataType=sfix(16)  OutScaling=2^0
  Gain2 : Gain  Gain=-1  ParameterDataType=sfix(16)  ParameterScaling=2^0  OutDataType=sfix(16)  OutScaling=2^0
  Gain3 : Gain  Gain=g*(m1*r1+m2*l1)  ParameterDataType=sfix(16)  ParameterScaling=2^0  OutDataType=sfix(16)  OutScaling=2^0
  Gain4 : Gain  Gain=m2*r2*g  ParameterDataType=sfix(16)  ParameterScaling=2^0  OutDataType=sfix(16)  OutScaling=2^0
  Gain5 : Gain  Gain=2  ParameterDataType=sfix(16)  ParameterScaling=2^0  OutDataType=sfix(16)  OutScaling=2^0
  Math Function : Math  Operator=magnitude^2  OutDataType=sfix(16)  OutScaling=2^0  SaturateOnIntegerOverflow=on
  Product : Product  OutDataType=sfix(16)  OutScaling=2^0  RndMeth=Zero
  Product1 : Product  OutDataType=sfix(16)  OutScaling=2^0  RndMeth=Zero
  Selector : Selector  InputPortWidth=4  IndexOptions=Index vector (dialog)  Indices=[1]  OutputSizes=1
  Selector1 : Selector  InputPortWidth=4  IndexOptions=Index vector (dialog)  Indices=[3]  OutputSizes=1
  Selector2 : Selector  InputPortWidth=4  IndexOptions=Index vector (dialog)  Indices=[2]  OutputSizes=1
  Selector3 : Selector  InputPortWidth=4  IndexOptions=Index vector (dialog)  Indices=[4]  OutputSizes=1
  Trigonometric Function : Trigonometry
  Trigonometric Function2 : Trigonometry  Operator=cos
  Trigonometric Function3 : Trigonometry  Operator=cos
  -F(1) : Outport  OutDataType=sfix(16)  OutScaling=2^0
  wires:
  Trigonometric Function/1 -> Gain1/1
  Selector1/1 -> Add1/2, Trigonometric Function/1  "x3"
  Selector/1 -> Add1/1, Trigonometric Function2/1  "x1"
  Trigonometric Function2/1 -> Gain3/1
  Gain3/1 -> Add/1
  Trigonometric Function3/1 -> Gain4/1  "cos(x1+x3)"
  Add1/1 -> Trigonometric Function3/1
  Gain4/1 -> Add/2
  Product1/1 -> Add/3  "x4^2*bsinx3"
  Add/1 -> Gain2/1
  x/1 -> Selector/1, Selector1/1, Selector2/1, Selector3/1
  Selector3/1 -> Product/2, Math Function/1  "x4"
  Selector2/1 -> Product/1  "x2"
  Math Function/1 -> Add2/2  "x4^2"
  Product/1 -> Gain5/1  "x2*x4"
  Gain5/1 -> Add2/1
  Add2/1 -> Product1/2
  Gain1/1 -> Product1/1
  Gain2/1 -> -F(1)/1

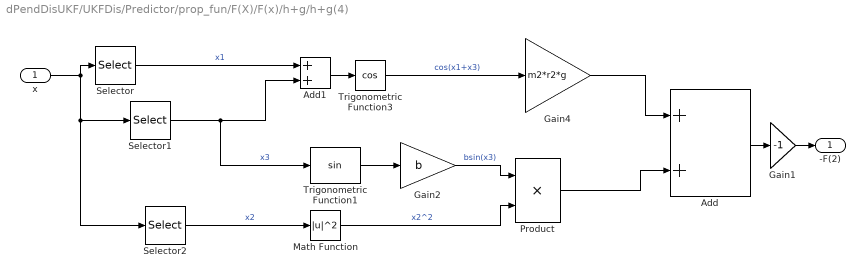
== system dPendDisUKF/UKFDis/Predictor/prop_fun/F(X)/F(x)/h+g/h+g(4) ==
  x : Inport
  Add : Sum  OutDataType=sfix(16)  OutScaling=2^-10
  Add1 : Sum  OutDataType=sfix(16)  OutScaling=2^-10
  Gain1 : Gain  Gain=-1  ParameterDataType=sfix(16)  ParameterScaling=2^0  OutDataType=sfix(16)  OutScaling=2^0
  Gain2 : Gain  Gain=b  ParameterDataType=sfix(16)  ParameterScaling=2^0  OutDataType=sfix(16)  OutScaling=2^0
  Gain4 : Gain  Gain=m2*r2*g  ParameterDataType=sfix(16)  ParameterScaling=2^0  OutDataType=sfix(16)  OutScaling=2^0
  Math Function : Math  Operator=magnitude^2  OutDataType=sfix(16)  OutScaling=2^0  SaturateOnIntegerOverflow=on
  Product : Product  OutDataType=sfix(16)  OutScaling=2^0  RndMeth=Zero
  Selector : Selector  InputPortWidth=4  IndexOptions=Index vector (dialog)  Indices=[1]  OutputSizes=1
  Selector1 : Selector  InputPortWidth=4  IndexOptions=Index vector (dialog)  Indices=[3]  OutputSizes=1
  Selector2 : Selector  InputPortWidth=4  IndexOptions=Index vector (dialog)  Indices=[2]  OutputSizes=1
  Trigonometric Function1 : Trigonometry
  Trigonometric Function3 : Trigonometry  Operator=cos
  -F(2) : Outport  OutDataType=sfix(16)  OutScaling=2^0
  wires:
  Selector2/1 -> Math Function/1  "x2"
  Product/1 -> Add/2
  Gain4/1 -> Add/1
  x/1 -> Selector/1, Selector1/1, Selector2/1
  Trigonometric Function1/1 -> Gain2/1
  Selector1/1 -> Trigonometric Function1/1, Add1/2  "x3"
  Selector/1 -> Add1/1  "x1"
  Trigonometric Function3/1 -> Gain4/1  "cos(x1+x3)"
  Add1/1 -> Trigonometric Function3/1
  Add/1 -> Gain1/1
  Gain2/1 -> Product/1  "bsin(x3)"
  Math Function/1 -> Product/2  "x2^2"
  Gain1/1 -> -F(2)/1

== system dPendDisUKF/UKFDis/Predictor/prop_fun/F(X)/F(x)/M matrix/M2/M22 ==
  x3 : Inport
  Constant : Constant  Value=a  OutDataType=sfix(16)  OutScaling=2^0
  Gain1 : Gain  Gain=2*b  ParameterDataType=sfix(16)  ParameterScaling=2^0  OutDataType=sfix(16)  OutScaling=2^0
  Sum : Sum  OutDataType=sfix(16)  OutScaling=2^0
  Trigonometric Function : Trigonometry  Operator=cos
  M22 : Outport
  wires:
  x3/1 -> Trigonometric Function/1
  Sum/1 -> M22/1  "a+2bCos(x3)"
  Gain1/1 -> Sum/2
  Trigonometric Function/1 -> Gain1/1
  Constant/1 -> Sum/1

== system dPendDisUKF/UKFDis/Predictor/prop_fun/F(X)/F(x)/M matrix/M2/M24 ==
  x3 : Inport
  Constant : Constant  Value=d  OutDataType=sfix(16)  OutScaling=2^0
  Gain1 : Gain  Gain=b  ParameterDataType=sfix(16)  ParameterScaling=2^0  OutDataType=sfix(16)  OutScaling=2^0
  Sum : Sum  OutDataType=sfix(16)  OutScaling=2^0
  Trigonometric Function : Trigonometry  Operator=cos
  M24 : Outport
  wires:
  Trigonometric Function/1 -> Gain1/1
  Gain1/1 -> Sum/2
  Sum/1 -> M24/1  "d+bCos(x3)"
  x3/1 -> Trigonometric Function/1
  Constant/1 -> Sum/1

== matlab function UKFDis/Predictor/Embedded MATLAB Function ==
  data: M input inherited; X output inherited; Pu input inherited; c input inherited
function X = ut_sigmas(M,Pu,c)

 A = chol(Pu)';

%{
  A = Pu;
  L  = zeros(size(A));
  def = 1;
  for i=1:size(A,1)
      for j=1:i
          s = A(i,j);
          for k=1:j-1
              s = s - L(i,k)*L(j,k);
          end
          if j < i
              if L(j,j) > eps
                  L(i,j) = s / L(j,j);
              else
                  L(i,j) = 0;
              end
          else
              if (s < -eps)
                  s = 0;
                  def = -1;
              elseif (s < eps)
                  s = 0;
                  def = min(0,def);
              end
              L(j,j) = sqrt(s);
          end
      end
  end
  A = L;
 %}
  X = [zeros(size(M)) A -A];
  X = sqrt(c)*X + repmat(M,1,size(X,2));

== matlab function UKFDis/Corrector/Embedded MATLAB Function ==
  data: M input inherited; X output inherited; Pu input inherited; c input inherited
function X = ut_sigmas(M,Pu,c)

A = chol(Pu)';

%{
  A = Pu;
  L  = zeros(size(A));
  def = 1;
  for i=1:size(A,1)
      for j=1:i
          s = A(i,j);
          for k=1:j-1
              s = s - L(i,k)*L(j,k);
          end
          if j < i
              if L(j,j) > eps
                  L(i,j) = s / L(j,j);
              else
                  L(i,j) = 0;
              end
          else
              if (s < -eps)
                  s = 0;
                  def = -1;
              elseif (s < eps)
                  s = 0;
                  def = min(0,def);
              end
              L(j,j) = sqrt(s);
          end
      end
  end
  A = L;
%}
  X = [zeros(size(M)) A -A];
  X = sqrt(c)*X + repmat(M,1,size(X,2));
